simulink model "EXPT8"  (R2021b)
settings: Solver=VariableStepAuto  StartTime=0.0  StopTime=200  RelTol=1e-3
libraries: simulink x1, spspowerguiLib x1
settings Model: PacingRate=1000  Creator=amans  LastModifiedBy=amans

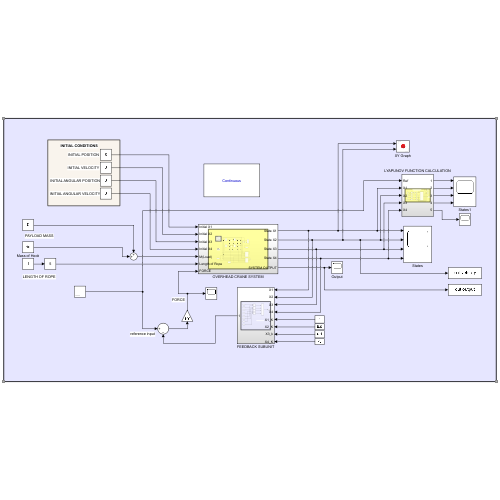
[thumbnail: Simulink's stored preview of the top-level diagram]
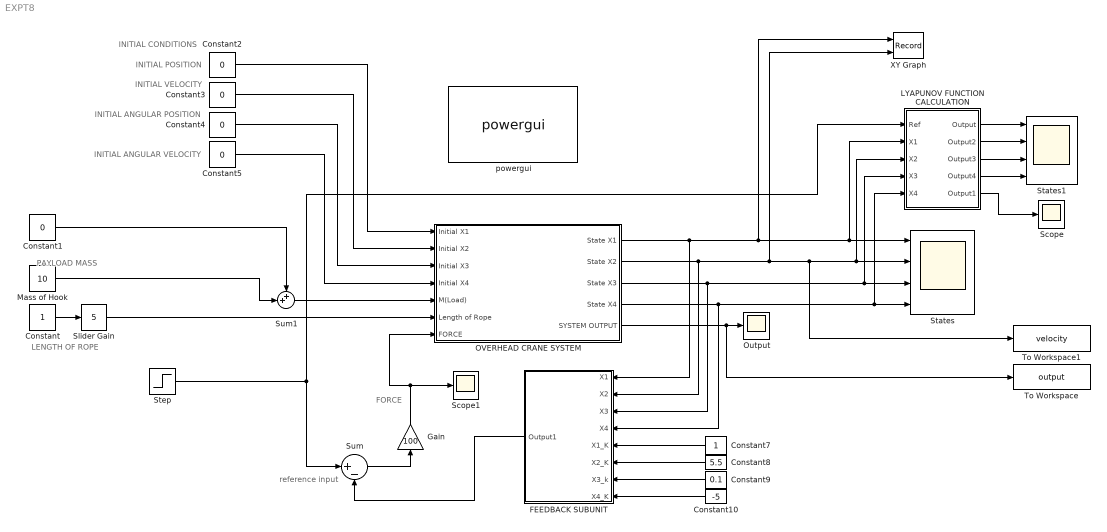
== system EXPT8 ==
  note: FORCE
  note: reference input
  note: LENGTH OF ROPE
  note: INITIAL ANGULAR VELOCITY
  note: INITIAL ANGULAR POSITION
  note: INITIAL VELOCITY
  note: INITIAL POSITION
  note: INITIAL CONDITIONS
  note: PAYLOAD MASS
  Constant : Constant
  Constant{1..5} (5 alike) : Constant  Value=0
  Constant10 : Constant  Value=-5
  Constant7 : Constant
  Constant8 : Constant  Value=5.5
  Constant9 : Constant  Value=0.1
  FEEDBACK SUBUNIT : Subsystem
  Gain : Gain  Gain=100
  LYAPUNOV FUNCTION CALCULATION : Subsystem
  Mass of Hook : Constant  Value=10
  OVERHEAD CRANE SYSTEM : Subsystem
  Output : Scope
  Scope : Scope
  Scope1 : Scope
  Slider Gain : simulink/Math Operations/Slider Gain  gain=5  low=1  high=25
  States : Scope  NumInputPorts=4
  States1 : Scope  NumInputPorts=4
  Step : Step  SampleTime=0
  Sum : Sum  Inputs=|+-
  Sum1 : Sum  Inputs=++|
  To Workspace : ToWorkspace  VariableName=output  SaveFormat=Timeseries  SampleTime=-1
  To Workspace1 : ToWorkspace  VariableName=velocity  SaveFormat=Timeseries  SampleTime=-1
  XY Graph : Record  FileSettingsInternal="{\"entries\":[{\"content\":{\"excelSettings\":{\"content\":{},\"type\":\"Streamout.ExcelSettings\"}},\"type\":\"Streamout.FileSettingStorage\",\"uuid\":\"c2f85f2e-b2fd-47b4-bf09-0d3d83d5f60a\"}],\"packageUris\":[\"http://schema.mathworks.com/mf0/streamout_blocks/R2020a\"],\"version\":\"1.0\"}"  Layout=[1 1]  SignalsInternal="{\"entries\":[{\"content\":{\"signals\":[{\"content\":{\"blockPath\":[\"EXPT8/XY Graph\"],\"channel\":[],\"dimensions\":[1],\"domain\":\"EXPT8/XY Graph\",\"lineColor\":\"#a2142f\",\"plots\":[1],\"port\":1,\"sid\":[],\"signalID\":9,\"signalName\":\"OVERHEAD CRANE SYSTEM:1\"},\"type\":\"RecordBlkView.Signal\",\"uuid\":\"2718287b-0875-4ae0-998d-ec136f265168\"},{\"content\":{\"blockPath\":[\"EXPT8/XY Graph\"],\"channel\":[],\"dimensions\":[1],\"domain\":\"EXPT8/XY Graph\",\"lineColor\":\"#139fff\",\"plots\":[1],\"port\":2,\"sid\":[],\"signalID\":12,\"signalName\":\"OVERHEAD CRANE SYSTEM:2\"},\"type\":\"RecordBlkView.Signal\",\"uuid\":\"42e2f042-69a5-4a3d-b452-4a78c1c86166\"}]},\"type\":\"RecordBlkView.InputSignals\",\"uuid\":\"803c249e-a84e-45e4-98e4-4698602c31aa\"}],\"packageUris\":[\"http://schema.mathworks.com/mf0/streamout_blocks/R2020a\"],\"version\":\"1.0\"}"  VisualizationBindings="{\"xyplotplugin\":{\"info\":[{\"series\":[{\"bindingParametersList\":[{\"parameter\":\"X-Axis\",\"signalID\":9,\"signalName\":\"OVERHEAD CRANE SYSTEM:1\"},{\"parameter\":\"Y-Axis\",\"signalID\":12,\"signalName\":\"OVERHEAD CRANE SYSTEM:2\"}],\"seriesID\":58305}],\"subplotID\":1}]}}"  CompatibilityTag=XY
  powergui : spspowerguiLib/powergui  Priority=1  SimulationMode=Continuous  SampleTime=50e-6  frequency=60  Iterations=50  frequencyindice=60  Pbase=100e6  ErrMax=1e-4  UnitsV=kV  UnitsW=MW  buscounter=0  FunctionMessages=off  echomessages=off  EnableUseOfTLC=off  CurrentSourceSwitches=off  DisableSnubberDevices=off  DisableRonSwitches=off  DisableVfSwitches=off  DisplayEquations=off  AutomaticDiscreteSolvers=off  SolverType=Tustin/Backward Euler (TBE)  Interpol=off  ExternalGateDelay=off  methode=off  Ts=100  x0status=blocks  SPID=on  SwTol=0  HookPort=off  NonlinearTolerance=1e-4  nMaxIteration=100  ContinueOnMaxIteration=off  RestoreLinks=warning  ResistiveCurrentMeasurement=off  Frange=[0:2:500]  Ylog=off  Xlog=on  ShowGrid=off  save=off  variable=ZData  structure=0  ZoomFFT=off  StartTime=0.0  cycles=1  DisplayStyle=1  fundamental=60  FreqAxis=off  MaxFrequency=1000  frequencyindicesteady=1  RmsSteady=1  display=off
  wires:
  Constant/1 -> Slider Gain/1
  OVERHEAD CRANE SYSTEM/2(State X2) -> FEEDBACK SUBUNIT/2(X2), XY Graph/2, To Workspace1/1, LYAPUNOV FUNCTION CALCULATION/3(X2), States/2
  OVERHEAD CRANE SYSTEM/3(State X3) -> FEEDBACK SUBUNIT/3(X3), LYAPUNOV FUNCTION CALCULATION/4(X3), States/3
  Constant2/1 -> OVERHEAD CRANE SYSTEM/1(Initial X1)
  Constant3/1 -> OVERHEAD CRANE SYSTEM/2(Initial X2)
  Constant4/1 -> OVERHEAD CRANE SYSTEM/3(Initial X3)
  Constant5/1 -> OVERHEAD CRANE SYSTEM/4(Initial X4)
  OVERHEAD CRANE SYSTEM/5(SYSTEM OUTPUT) -> Output/1, To Workspace/1
  OVERHEAD CRANE SYSTEM/1(State X1) -> FEEDBACK SUBUNIT/1(X1), XY Graph/1, LYAPUNOV FUNCTION CALCULATION/2(X1), States/1
  Slider Gain/1 -> OVERHEAD CRANE SYSTEM/6(Length of Rope)
  Constant1/1 -> Sum1/1
  Mass of Hook/1 -> Sum1/2
  Sum1/1 -> OVERHEAD CRANE SYSTEM/5(M(Load))
  OVERHEAD CRANE SYSTEM/4(State X4) -> LYAPUNOV FUNCTION CALCULATION/5(X4), States/4, FEEDBACK SUBUNIT/4(X4)
  LYAPUNOV FUNCTION CALCULATION/5(Output1) -> Scope/1
  Sum/1 -> Gain/1
  Constant7/1 -> FEEDBACK SUBUNIT/5(X1_K)
  Constant8/1 -> FEEDBACK SUBUNIT/6(X2_K)
  Constant9/1 -> FEEDBACK SUBUNIT/7(X3_k)
  Constant10/1 -> FEEDBACK SUBUNIT/8(X4_K)
  Step/1 -> Sum/1, LYAPUNOV FUNCTION CALCULATION/1(Ref)
  LYAPUNOV FUNCTION CALCULATION/1(Output) -> States1/1
  LYAPUNOV FUNCTION CALCULATION/2(Output2) -> States1/2
  LYAPUNOV FUNCTION CALCULATION/3(Output3) -> States1/3
  LYAPUNOV FUNCTION CALCULATION/4(Output4) -> States1/4
  FEEDBACK SUBUNIT/1(Output1) -> Sum/2
  Gain/1 -> OVERHEAD CRANE SYSTEM/7(FORCE), Scope1/1

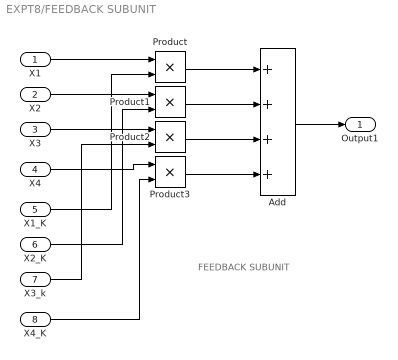
== system EXPT8/FEEDBACK SUBUNIT ==
  note: FEEDBACK SUBUNIT
  X1 : Inport
  X2 : Inport  Port=2
  X3 : Inport  Port=3
  X4 : Inport  Port=4
  X1_K : Inport  Port=5
  X2_K : Inport  Port=6
  X3_k : Inport  Port=7
  X4_K : Inport  Port=8
  Add : Sum  Inputs=++++
  Product{,1..3} (4 alike) : Product
  Output1 : Outport
  wires:
  Product2/1 -> Add/3
  X1/1 -> Product/1
  X3_k/1 -> Product2/2
  X4/1 -> Product3/1
  X2_K/1 -> Product1/2
  Product/1 -> Add/1
  X1_K/1 -> Product/2
  X3/1 -> Product2/1
  Add/1 -> Output1/1
  X4_K/1 -> Product3/2
  X2/1 -> Product1/1
  Product1/1 -> Add/2
  Product3/1 -> Add/4

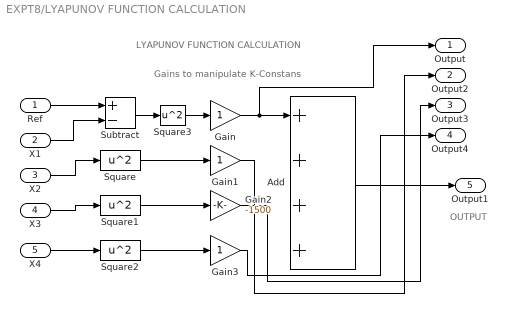
== system EXPT8/LYAPUNOV FUNCTION CALCULATION ==
  note: OUTPUT
  note: LYAPUNOV FUNCTION CALCULATION
  note: Gains to manipulate K-Constans
  Ref : Inport
  X1 : Inport  Port=2
  X2 : Inport  Port=3
  X3 : Inport  Port=4
  X4 : Inport  Port=5
  Add : Sum  Inputs=++++
  Gain : Gain
  Gain1 : Gain
  Gain2 : Gain  Gain=-1500
  Gain3 : Gain
  Square{,1..3} (4 alike) : Math  Operator=square  SaturateOnIntegerOverflow=on
  Subtract : Sum  Inputs=+-
  Output : Outport
  Output2 : Outport  Port=2
  Output3 : Outport  Port=3
  Output4 : Outport  Port=4
  Output1 : Outport  Port=5
  wires:
  X1/1 -> Subtract/2
  X3/1 -> Square1/1
  X4/1 -> Square2/1
  Subtract/1 -> Square3/1
  Add/1 -> Output1/1
  X2/1 -> Square/1
  Ref/1 -> Subtract/1
  Square3/1 -> Gain/1
  Square/1 -> Gain1/1
  Square1/1 -> Gain2/1
  Square2/1 -> Gain3/1
  Gain/1 -> Output/1, Add/1
  Gain1/1 -> Output2/1
  Gain3/1 -> Output4/1
  Gain2/1 -> Output3/1

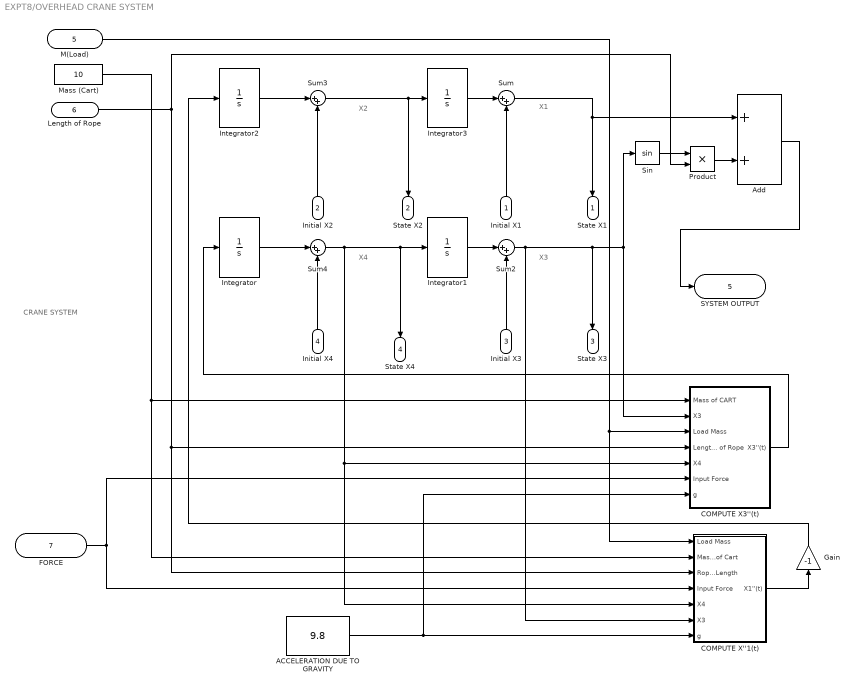
== system EXPT8/OVERHEAD CRANE SYSTEM ==
  note: CRANE SYSTEM
  note: X3
  note: X4
  note: X1
  note: X2
  Initial X1 : Inport
  Initial X2 : Inport  Port=2
  Initial X3 : Inport  Port=3
  Initial X4 : Inport  Port=4
  M(Load) : Inport  Port=5
  Length of Rope : Inport  Port=6
  FORCE : Inport  Port=7
  ACCELERATION DUE TO GRAVITY : Constant  Value=9.8
  Add : Sum
  COMPUTE X''1(t) : Subsystem
  COMPUTE X3''(t) : Subsystem
  Gain : Gain  Gain=-1
  Integrator{,1..3} (4 alike) : Integrator
  Mass (Cart) : Constant  Value=10
  Product : Product
  Sin : Trigonometry
  Sum{,2..4} (4 alike) : Sum  Inputs=|++
  State X1 : Outport
  State X2 : Outport  Port=2
  State X3 : Outport  Port=3
  State X4 : Outport  Port=4
  SYSTEM OUTPUT : Outport  Port=5
  wires:
  Sin/1 -> Product/1
  Initial X2/1 -> Sum3/2
  M(Load)/1 -> COMPUTE X''1(t)/1(Load Mass), COMPUTE X3''(t)/3(Load Mass)
  Sum3/1 -> State X2/1, Integrator3/1
  Length of Rope/1 -> Product/2, COMPUTE X''1(t)/3(Rope Length), COMPUTE X3''(t)/4(Length of Rope)
  Sum2/1 -> COMPUTE X''1(t)/6(X3), State X3/1, COMPUTE X3''(t)/2(X3), Sin/1
  COMPUTE X''1(t)/1(X1''(t)) -> Gain/1
  COMPUTE X3''(t)/1(X3''(t)) -> Integrator/1
  FORCE/1 -> COMPUTE X3''(t)/6(Input Force), COMPUTE X''1(t)/4(Input Force)
  ACCELERATION DUE TO GRAVITY/1 -> COMPUTE X3''(t)/7(g), COMPUTE X''1(t)/7(g)
  Sum4/1 -> COMPUTE X''1(t)/5(X4), COMPUTE X3''(t)/5(X4), State X4/1, Integrator1/1
  Product/1 -> Add/2
  Integrator1/1 -> Sum2/1
  Mass (Cart)/1 -> COMPUTE X''1(t)/2(Mass of Cart), COMPUTE X3''(t)/1(Mass of CART)
  Integrator3/1 -> Sum/1
  Initial X4/1 -> Sum4/2
  Integrator2/1 -> Sum3/1
  Integrator/1 -> Sum4/1
  Initial X1/1 -> Sum/2
  Initial X3/1 -> Sum2/2
  Sum/1 -> State X1/1, Add/1
  Add/1 -> SYSTEM OUTPUT/1
  Gain/1 -> Integrator2/1

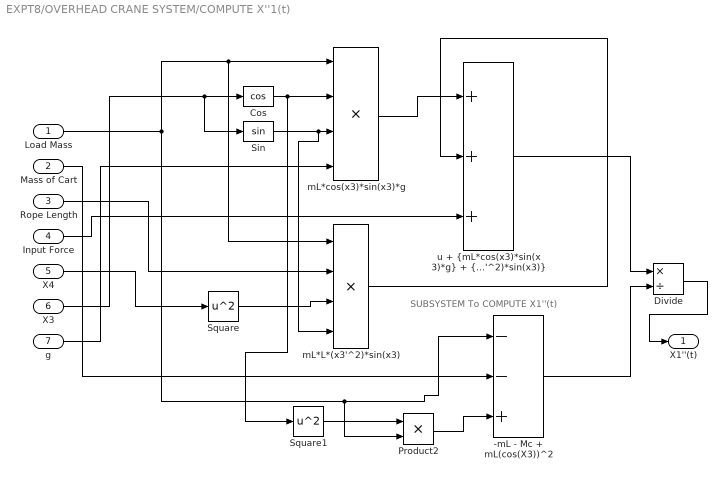
== system EXPT8/OVERHEAD CRANE SYSTEM/COMPUTE X''1(t) ==
  note: SUBSYSTEM To COMPUTE X1''(t)
  Load Mass : Inport
  Mass of Cart : Inport  Port=2
  Rope Length : Inport  Port=3
  Input Force : Inport  Port=4
  X4 : Inport  Port=5
  X3 : Inport  Port=6
  g : Inport  Port=7
  -mL - Mc + mL(cos(X3))^2 : Sum  Inputs=--+
  Cos : Trigonometry  Operator=cos
  Divide : Product  Inputs=*/
  Product2 : Product
  Sin : Trigonometry
  Square : Math  Operator=square  SaturateOnIntegerOverflow=on
  Square1 : Math  Operator=square  SaturateOnIntegerOverflow=on
  mL*L*(x3'^2)*sin(x3) : Product  Inputs=4
  mL*cos(x3)*sin(x3)*g : Product  Inputs=4
  "u + {mL*cos(x3)*sin(x3)*g} + {mL*L*(x3'^2)*sin(x3)} " : Sum  Inputs=+++
  X1''(t) : Outport
  wires:
  "u + {mL*cos(x3)*sin(x3)*g} + {mL*L*(x3'^2)*sin(x3)} "/1 -> Divide/1
  Load Mass/1 -> mL*L*(x3'^2)*sin(x3)/1, mL*cos(x3)*sin(x3)*g/1, -mL - Mc + mL(cos(X3))^2/1, Product2/2
  Sin/1 -> mL*L*(x3'^2)*sin(x3)/4, mL*cos(x3)*sin(x3)*g/3
  Cos/1 -> Square1/1, mL*cos(x3)*sin(x3)*g/2
  Square/1 -> mL*L*(x3'^2)*sin(x3)/3
  Product2/1 -> -mL - Mc + mL(cos(X3))^2/3
  X3/1 -> Sin/1, Cos/1
  Square1/1 -> Product2/1
  mL*L*(x3'^2)*sin(x3)/1 -> "u + {mL*cos(x3)*sin(x3)*g} + {mL*L*(x3'^2)*sin(x3)} "/2
  mL*cos(x3)*sin(x3)*g/1 -> "u + {mL*cos(x3)*sin(x3)*g} + {mL*L*(x3'^2)*sin(x3)} "/1
  -mL - Mc + mL(cos(X3))^2/1 -> Divide/2
  Divide/1 -> X1''(t)/1
  Input Force/1 -> "u + {mL*cos(x3)*sin(x3)*g} + {mL*L*(x3'^2)*sin(x3)} "/3
  Rope Length/1 -> mL*L*(x3'^2)*sin(x3)/2
  Mass of Cart/1 -> -mL - Mc + mL(cos(X3))^2/2
  g/1 -> mL*cos(x3)*sin(x3)*g/4
  X4/1 -> Square/1

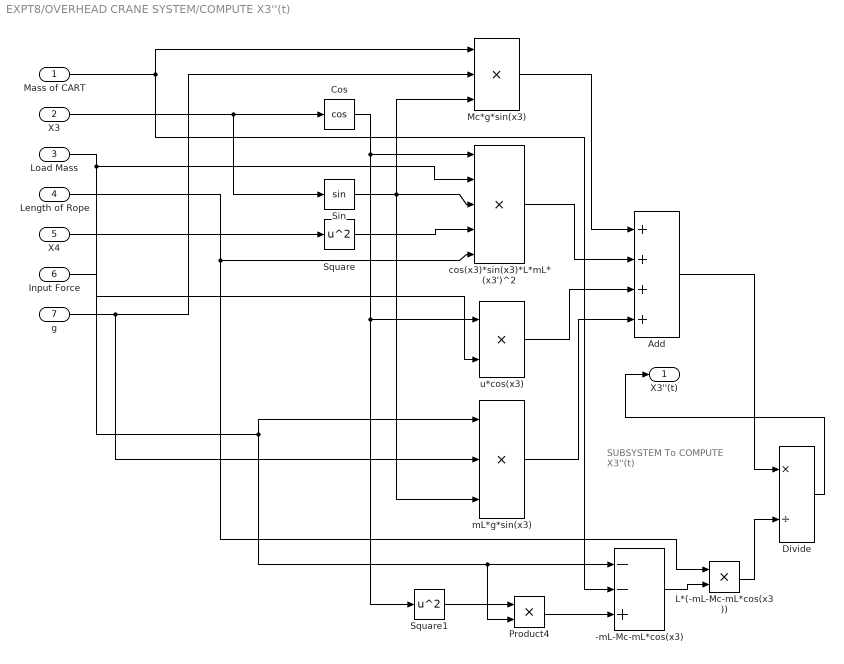
== system EXPT8/OVERHEAD CRANE SYSTEM/COMPUTE X3''(t) ==
  note: SUBSYSTEM To COMPUTE X3''(t)
  Mass of CART : Inport
  X3 : Inport  Port=2
  Load Mass : Inport  Port=3
  Length of Rope : Inport  Port=4
  X4 : Inport  Port=5
  Input Force : Inport  Port=6
  g : Inport  Port=7
  -mL-Mc-mL*cos(x3) : Sum  Inputs=--+
  Add : Sum  Inputs=++++
  Cos : Trigonometry  Operator=cos
  Divide : Product  Inputs=*/
  L*(-mL-Mc-mL*cos(x3)) : Product
  Mc*g*sin(x3) : Product  Inputs=3
  Product4 : Product
  Sin : Trigonometry
  Square : Math  Operator=square  SaturateOnIntegerOverflow=on
  Square1 : Math  Operator=square  SaturateOnIntegerOverflow=on
  cos(x3)*sin(x3)*L*mL*(x3')^2 : Product  Inputs=5
  mL*g*sin(x3) : Product  Inputs=3
  u*cos(x3) : Product
  X3''(t) : Outport
  wires:
  Length of Rope/1 -> L*(-mL-Mc-mL*cos(x3))/1, cos(x3)*sin(x3)*L*mL*(x3')^2/5
  Mc*g*sin(x3)/1 -> Add/1
  u*cos(x3)/1 -> Add/3
  Load Mass/1 -> Product4/2, -mL-Mc-mL*cos(x3)/1, mL*g*sin(x3)/1, cos(x3)*sin(x3)*L*mL*(x3')^2/2
  cos(x3)*sin(x3)*L*mL*(x3')^2/1 -> Add/2
  Cos/1 -> Square1/1, u*cos(x3)/1, cos(x3)*sin(x3)*L*mL*(x3')^2/1
  g/1 -> mL*g*sin(x3)/2, Mc*g*sin(x3)/2
  Mass of CART/1 -> Mc*g*sin(x3)/1, -mL-Mc-mL*cos(x3)/2
  Sin/1 -> mL*g*sin(x3)/3, cos(x3)*sin(x3)*L*mL*(x3')^2/3, Mc*g*sin(x3)/3
  X3/1 -> Cos/1, Sin/1
  Add/1 -> Divide/1
  L*(-mL-Mc-mL*cos(x3))/1 -> Divide/2
  -mL-Mc-mL*cos(x3)/1 -> L*(-mL-Mc-mL*cos(x3))/2
  Square/1 -> cos(x3)*sin(x3)*L*mL*(x3')^2/4
  Square1/1 -> Product4/1
  Product4/1 -> -mL-Mc-mL*cos(x3)/3
  mL*g*sin(x3)/1 -> Add/4
  Input Force/1 -> u*cos(x3)/2
  X4/1 -> Square/1
  Divide/1 -> X3''(t)/1
